simulink model "ThreePhaseControlledConveter"  (R2024a)
settings: Solver=VariableStepAuto  StartTime=0.0  StopTime=0.1  RelTol=1e-3
libraries: spsThyristorLib x6, spsCurrentMeasurementLib x2, spsVoltageMeasurementLib x2, spsDCVoltageSourceLib x1, spsGroundLib x1, spsSeriesRLCBranchLib x1, spsThreePhaseProgrammableVoltageSourceLib x1, sps_lib x1
settings Model: Creator=danielmcguiness  LastModifiedBy=danielmcguiness

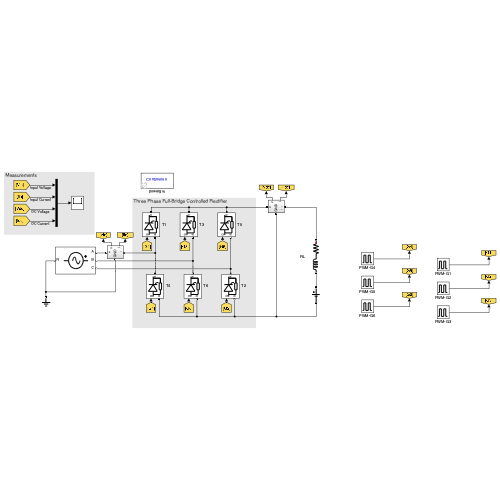
[thumbnail: Simulink's stored preview of the top-level diagram]
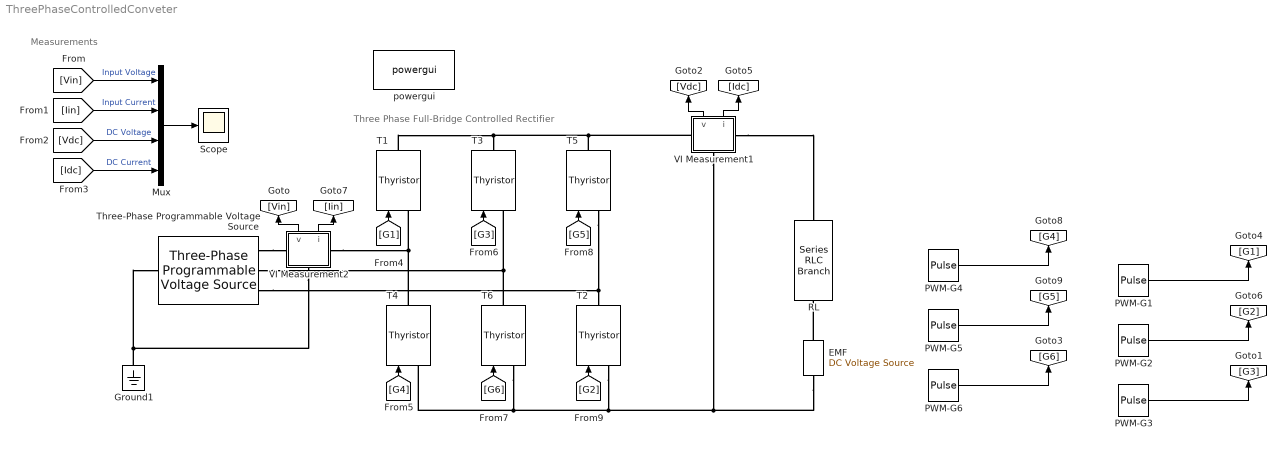
== system ThreePhaseControlledConveter ==
  note: Measurements
  note: Three Phase Full-Bridge Controlled Rectifier
  EMF : spsDCVoltageSourceLib/DC Voltage Source  Amplitude=50  Measurements=None
  Ground1 : spsGroundLib/Ground  LConnTagsString=a
  Mux : Mux
  PWM-G1 : DiscretePulseGenerator  PulseType=Time based  Amplitude=100  Period=1/50  PulseWidth=50  PhaseDelay=(1/50) * (45/360)
  PWM-G2 : DiscretePulseGenerator  PulseType=Time based  Amplitude=100  Period=1/50  PulseWidth=50  PhaseDelay=(1/50) * ((45/360) + 60/360)
  PWM-G3 : DiscretePulseGenerator  PulseType=Time based  Amplitude=100  Period=1/50  PulseWidth=50  PhaseDelay=(1/50) * ((45/360) + 120/360)
  PWM-G4 : DiscretePulseGenerator  PulseType=Time based  Amplitude=100  Period=1/50  PulseWidth=50  PhaseDelay=(1/50) * ((45/360)+ 0.5)
  PWM-G5 : DiscretePulseGenerator  PulseType=Time based  Amplitude=100  Period=1/50  PulseWidth=50  PhaseDelay=(1/50) * ((45/360) + 60/360 + 0.5)
  PWM-G6 : DiscretePulseGenerator  PulseType=Time based  Amplitude=100  Period=1/50  PulseWidth=50  PhaseDelay=(1/50) * ((45/360) + 120/360 + 0.5)
  RL : spsSeriesRLCBranchLib/Series RLC Branch  LConnTagsString=__new0  RConnTagsString=__new0  BranchType=RL  Resistance=1  Inductance=20e-3  SetiL0=off  InitialCurrent=0  Capacitance=1e-6  Setx0=off  InitialVoltage=0  Measurements=None
  Scope : Scope
  T{1..6} (6 alike) : spsThyristorLib/Thyristor  Ron=0.001  Lon=0  Vf=0.8  IC=0  Rs=500  Cs=250e-9  Measurements=off
  Three-Phase Programmable Voltage Source : spsThreePhaseProgrammableVoltageSourceLib/Three-Phase Programmable Voltage Source  PositiveSequence="[100  0 50]"  VariationEntity=None  VariationType=Table of time-amplitude pairs  VariationTypeAlt=Step  VariationStep=0.5  VariationRate=10  VariationMagnitude=0.3  VariationFrequency=2  VariationTiming=[1 2]  VariationPhaseA=off  Amplitudes=[1 0.8 1.2 1.0]  TimeValues=[0 0.1 0.15 0.2]  HarmonicGeneration=off  HarmonicA=[3 0.2 -25 0]  HarmonicB=[2 0.15 35 2]  Timing="[0.05  3]"  BusType=swing  Pref=0  Qref=0  Qmin=-inf  Qmax=inf
  VI Measurement1 : Subsystem
      settings: PortSchema="{\"entries\":[{\"content\":{\"sides\":[{\"content\":{\"connectorIds\":[\"LConn1\"]},\"type\":\"ConnectorPlacement.EquallySpacedRectSide\",\"uuid\":\"d0d06b58-e7a6-4090-bc4f-be16d4258115\"},{\"content\":{\"connectorIds\":[\"RConn1\"],\"side\":\"RIGHT\"},\"type\":\"ConnectorPlacement.EquallySpacedRectSide\",\"uuid\":\"ec0e199e-bf94-46e5-8fb5-fcfe43c2f9e8\"},{\"content\":{\"connectorIds\":[\"Out1\",\"Out2\"],\"side\":\"TOP\"},\"type\":\"ConnectorPlacement.EquallySpacedRectSide\",\"uuid\":\"e633db83-a48d-4359-b0a8-630d80fecfae\"},{\"content\":{\"connectorIds\":[\"RConn2\"],\"side\":\"BOTTOM\"},\"type\":\"ConnectorPlacement.EquallySpacedRectSide\",\"uuid\":\"46b0a315-b5ae-4457-83c3-69b7a744a381\"}]},\"type\":\"ConnectorPlacement.EquallySpacedConnector\",\"uuid\":\"3aa23921-cdab-42f2-9dd1-6188dd33585f\"}],\"packageUris\":[\"http://schema.mathworks.com/mf0/Connector/R2020b\"],\"version\":\"1.0\"}"
  VI Measurement2 : Subsystem
      settings: PortSchema="{\"entries\":[{\"content\":{\"sides\":[{\"content\":{\"connectorIds\":[\"LConn1\"]},\"type\":\"ConnectorPlacement.EquallySpacedRectSide\",\"uuid\":\"d0d06b58-e7a6-4090-bc4f-be16d4258115\"},{\"content\":{\"connectorIds\":[\"RConn1\"],\"side\":\"RIGHT\"},\"type\":\"ConnectorPlacement.EquallySpacedRectSide\",\"uuid\":\"ec0e199e-bf94-46e5-8fb5-fcfe43c2f9e8\"},{\"content\":{\"connectorIds\":[\"Out1\",\"Out2\"],\"side\":\"TOP\"},\"type\":\"ConnectorPlacement.EquallySpacedRectSide\",\"uuid\":\"e633db83-a48d-4359-b0a8-630d80fecfae\"},{\"content\":{\"connectorIds\":[\"RConn2\"],\"side\":\"BOTTOM\"},\"type\":\"ConnectorPlacement.EquallySpacedRectSide\",\"uuid\":\"46b0a315-b5ae-4457-83c3-69b7a744a381\"}]},\"type\":\"ConnectorPlacement.EquallySpacedConnector\",\"uuid\":\"3aa23921-cdab-42f2-9dd1-6188dd33585f\"}],\"packageUris\":[\"http://schema.mathworks.com/mf0/Connector/R2020b\"],\"version\":\"1.0\"}"
  powergui : sps_lib/powergui  Priority=1  SimulationMode=Continuous  SampleTime=50e-6  frequency=60  Iterations=50  frequencyindice=50  Pbase=100e6  ErrMax=1e-4  UnitsV=kV  UnitsW=MW  buscounter=0  FunctionMessages=off  echomessages=off  EnableUseOfTLC=off  CurrentSourceSwitches=off  DisableSnubberDevices=off  DisableRonSwitches=off  DisableVfSwitches=off  DisplayEquations=off  AutomaticDiscreteSolvers=off  SolverType=Tustin/Backward Euler (TBE)  Interpol=off  ExternalGateDelay=off  methode=off  Ts=100  x0status=blocks  SPID=on  SwTol=0  HookPort=off  NonlinearTolerance=1e-4  nMaxIteration=100  ContinueOnMaxIteration=off  RestoreLinks=warning  ResistiveCurrentMeasurement=off  Frange=[0:2:500]  Ylog=off  Xlog=on  ShowGrid=off  save=off  variable=ZData  structure=0  ZoomFFT=off  StartTime=0.0  cycles=1  DisplayStyle=1  fundamental=60  FreqAxis=off  MaxFrequency=1000  frequencyindicesteady=1  RmsSteady=1  display=off
  wires:
  Mux/1 -> Scope/1
  [Vdc] -> Mux/3  "DC Voltage"
  [G1] -> T1/1
  [G4] -> T4/1
  [G3] -> T3/1
  [G6] -> T6/1
  [Idc] -> Mux/4  "DC Current"
  [Iin] -> Mux/2  "Input Current"
  [Vin] -> Mux/1  "Input Voltage"
  [G5] -> T5/1
  [G2] -> T2/1
  VI Measurement1/1(v) -> [Vdc]
  VI Measurement1/2(i) -> [Idc]
  VI Measurement2/1(v) -> [Vin]
  VI Measurement2/2(i) -> [Iin]
  PWM-G5/1 -> [G5]
  PWM-G1/1 -> [G1]
  PWM-G3/1 -> [G3]
  PWM-G6/1 -> [G6]
  PWM-G4/1 -> [G4]
  PWM-G2/1 -> [G2]
  connections:
  T4/RConn1 -- VI Measurement2/RConn1 -- T1/LConn1
  T1/RConn1 -- VI Measurement1/LConn1 -- T5/RConn1 -- T3/RConn1
  T6/LConn1 -- EMF/LConn1 -- VI Measurement1/RConn2 -- T2/LConn1 -- T4/LConn1
  T6/RConn1 -- Three-Phase Programmable Voltage Source/RConn2 -- T3/LConn1
  EMF/RConn1 -- RL/RConn1
  Ground1/LConn1 -- VI Measurement2/RConn2 -- Three-Phase Programmable Voltage Source/LConn1
  T5/LConn1 -- Three-Phase Programmable Voltage Source/RConn3 -- T2/RConn1
  VI Measurement1/RConn1 -- RL/LConn1
  Three-Phase Programmable Voltage Source/RConn1 -- VI Measurement2/LConn1

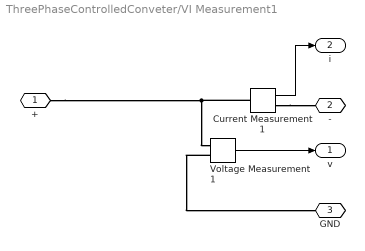
== system ThreePhaseControlledConveter/VI Measurement1 ==
  Current Measurement1 : spsCurrentMeasurementLib/Current Measurement  PhasorSimulation=off  OutputType=Complex  PSBequivalent=0
  Voltage Measurement1 : spsVoltageMeasurementLib/Voltage Measurement  PhasorSimulation=off  OutputType=Complex  PSBequivalent=0
  + : PMIOPort  Side=Left
  - : PMIOPort  Port=2  Side=Right
  GND : PMIOPort  Port=3  Side=Right
  v : Outport
  i : Outport  Port=2
  wires:
  Voltage Measurement1/1 -> v/1
  Current Measurement1/1 -> i/1
  connections:
  Current Measurement1/LConn1 -- Voltage Measurement1/LConn1 -- +/RConn1
  Voltage Measurement1/LConn2 -- GND/RConn1
  Current Measurement1/RConn1 -- -/RConn1

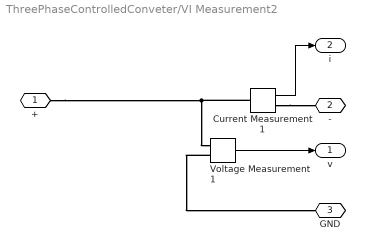
== system ThreePhaseControlledConveter/VI Measurement2 ==
  Current Measurement1 : spsCurrentMeasurementLib/Current Measurement  PhasorSimulation=off  OutputType=Complex  PSBequivalent=0
  Voltage Measurement1 : spsVoltageMeasurementLib/Voltage Measurement  PhasorSimulation=off  OutputType=Complex  PSBequivalent=0
  + : PMIOPort  Side=Left
  - : PMIOPort  Port=2  Side=Right
  GND : PMIOPort  Port=3  Side=Right
  v : Outport
  i : Outport  Port=2
  wires:
  Voltage Measurement1/1 -> v/1
  Current Measurement1/1 -> i/1
  connections:
  Current Measurement1/LConn1 -- Voltage Measurement1/LConn1 -- +/RConn1
  Voltage Measurement1/LConn2 -- GND/RConn1
  Current Measurement1/RConn1 -- -/RConn1
